simulink library "v2x_modem"  (R2021b)
settings: Solver=VariableStepAuto  StartTime=0.0  StopTime=10.0  RelTol=1e-3
libraries: commsync2 x3, commrfcorlib x2, commfilt2 x2, dspstat3 x1, commrflib2 x1
settings Model: Creator=jacob  LastModifiedBy=jacob

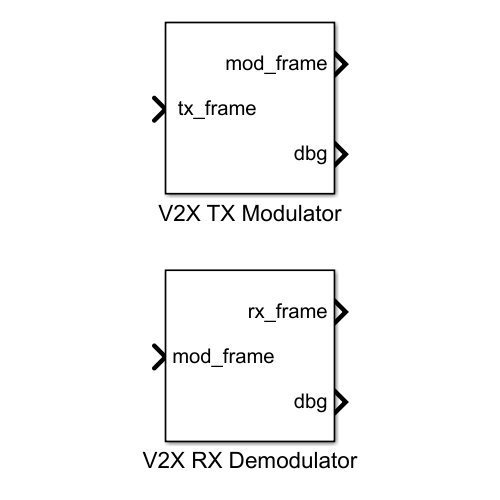
[thumbnail: Simulink's stored preview of the top-level diagram]
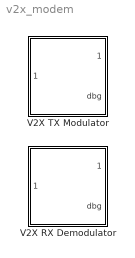
== system v2x_modem ==
  V2X RX Demodulator : Subsystem
      mask init:
      | ini = v2x_modem_init();
  V2X TX Modulator : Subsystem
      mask init:
      | ini = v2x_modem_init();

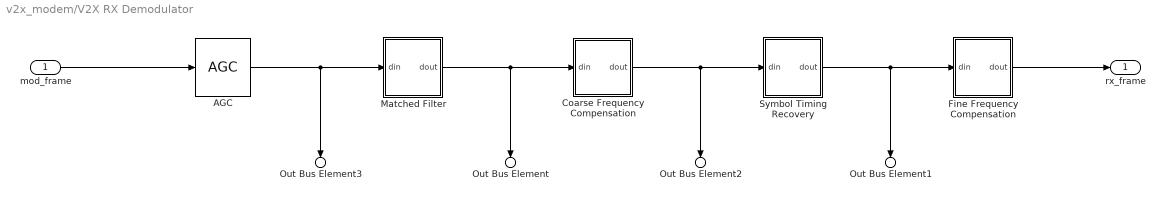
== system v2x_modem/V2X RX Demodulator ==
  mod_frame : Inport
  AGC : commrfcorlib/AGC  LegacyMode=off  DetectorMethod=Rectifier  LoopMethod=Linear  UpdatePeriod=100  StepSize=0.1  AdaptationStepSize=ini.agc_params.step_size  DesiredOutputPower=ini.agc_params.desired_out_pwr  AveragingLength=ini.agc_params.avg_len  MaximumGain=30  MaxPowerGain=ini.agc_params.max_gain_dB  GainOutputPort=off  InputPowerOutputPort=off  SimulateUsing=Interpreted execution
  Coarse Frequency Compensation : Subsystem
  Fine Frequency Compensation : Subsystem
  Matched Filter : Subsystem
  Symbol Timing Recovery : Subsystem
  rx_frame : Outport
  Out Bus Element3 : Outport  Port=2  PortName=dbg  Element=agc_out
  Out Bus Element : Outport  Port=2  PortName=dbg  Element=mf_out
  Out Bus Element2 : Outport  Port=2  PortName=dbg  Element=cfc_out
  Out Bus Element1 : Outport  Port=2  PortName=dbg  Element=str_out
  wires:
  AGC/1 -> Matched Filter/1(din), Out Bus Element3/1
  Coarse Frequency Compensation/1(dout) -> Out Bus Element2/1, Symbol Timing Recovery/1(din)
  Fine Frequency Compensation/1(dout) -> rx_frame/1
  Symbol Timing Recovery/1(dout) -> Out Bus Element1/1, Fine Frequency Compensation/1(din)
  Matched Filter/1(dout) -> Coarse Frequency Compensation/1(din), Out Bus Element/1
  mod_frame/1 -> AGC/1

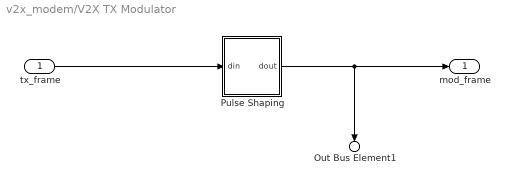
== system v2x_modem/V2X TX Modulator ==
  " tx_frame" : Inport
  Pulse Shaping : Subsystem
  mod_frame : Outport
  Out Bus Element1 : Outport  Port=2  PortName=dbg  Element=ps_out
  wires:
  " tx_frame"/1 -> Pulse Shaping/1(din)
  Pulse Shaping/1(dout) -> Out Bus Element1/1, mod_frame/1

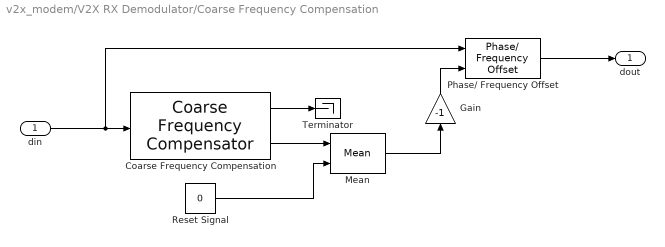
== system v2x_modem/V2X RX Demodulator/Coarse Frequency Compensation ==
  din : Inport
  Coarse Frequency Compensation : commrfcorlib/Coarse Frequency Compensator  Modulation=QPSK  Algorithm=Correlation-based  FrequencyResolution=25  MaximumFrequencyOffset=ini.freq_params.max_fo  SamplesPerSymbol=4  EstimatedFreqOffsetPort=on  SimulateUsing=Code generation
      settings: SourceProductBaseCode=CM
  Gain : Gain  Gain=-1
  Mean : dspstat3/Mean  run=on  InputProcessing=Columns as channels (frame based)  reset_popup=Either edge  directionMode=Each column  dimension=1  roiEnable=off  roiType=Rectangles  roiPortion=Entire ROI  roiOutput=Individual statistics for each ROI  roiFlag=off  roundingMode=Floor  overflowMode=off  outputDataTypeStr=Inherit: Same as accumulator  outputMin=[]  outputMax=[]  outputLastDataTypeStr=Inherit: Same as accumulator
  Phase/ Frequency Offset : commrflib2/Phase// Frequency Offset  phaseOffset=0  freqPort=on  freqOffset=0
  Reset Signal : Constant  Value=0  SampleTime=-1
  Terminator : Terminator
  dout : Outport  VectorParamsAs1DForOutWhenUnconnected=off
  wires:
  Reset Signal/1 -> Mean/2
  Gain/1 -> Phase/ Frequency Offset/2
  Coarse Frequency Compensation/1 -> Terminator/1
  Coarse Frequency Compensation/2 -> Mean/1
  Mean/1 -> Gain/1
  Phase/ Frequency Offset/1 -> dout/1
  din/1 -> Coarse Frequency Compensation/1, Phase/ Frequency Offset/1

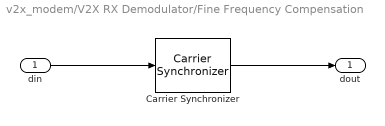
== system v2x_modem/V2X RX Demodulator/Fine Frequency Compensation ==
  din : Inport
  Carrier Synchronizer : commsync2/Carrier Synchronizer  Modulation=QPSK  ModulationPhaseOffset=Auto  CustomPhaseOffset=0  SamplesPerSymbol=ini.srrc_params.sps  DampingFactor=ini.timing_recov_params.damping_fact  NormalizedLoopBandwidth=ini.timing_recov_params.norm_loop_bw  EstimatedPhaseErrorOutputPort=off  SimulateUsing=Code generation
  dout : Outport
  wires:
  Carrier Synchronizer/1 -> dout/1
  din/1 -> Carrier Synchronizer/1

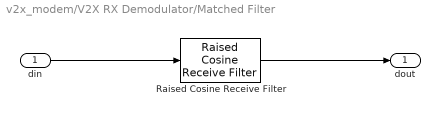
== system v2x_modem/V2X RX Demodulator/Matched Filter ==
  din : Inport
  Raised Cosine Receive Filter : commfilt2/Raised Cosine Receive Filter  filtType=Square root  R=ini.srrc_params.rolloff  filtSpan=ini.srrc_params.filt_span  N=ini.srrc_params.sps  downFactor=ini.srrc_params.decim  downOffset=0  filterGain=ini.srrc_params.lin_amp  InputProcessing=Columns as channels (frame based)  RateOptions=Allow multirate processing  framing=Mute  checkCoeff=off  variableName=rcRxFilt  currentFiltSpan=10  D=5  inputOffset=0  sampMode=Mute  saveAsFlag=0  rateMode=Downsampling  checkGain=Normalized  launchFVT=on  roundingMode=Floor  overflowMode=off  coeffDataTypeStr=Inherit: Same word length as input  coeffMin=[]  coeffMax=[]  coeffLastDataTypeStr=Inherit: Same word length as input  accumDataTypeStr=Inherit: Same as product output  accumLastDataTypeStr=Inherit: Same as product output  outputDataTypeStr=Inherit: Same as accumulator  outputMin=[]  outputMax=[]  outputLastDataTypeStr=Inherit: Same as accumulator
  dout : Outport
  wires:
  Raised Cosine Receive Filter/1 -> dout/1
  din/1 -> Raised Cosine Receive Filter/1

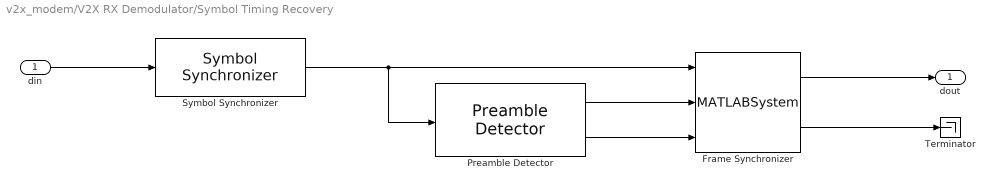
== system v2x_modem/V2X RX Demodulator/Symbol Timing Recovery ==
  din : Inport
  Frame Synchronizer : MATLABSystem  System=FrameSynchronizer  Input=Symbol  OutputFrameLength=ini.bb.intfc_params.tx_frame_len  PreambleLength=ini.bb.preamble_params.len  SimulateUsing=Code generation
      mask Type: FrameSynchronizer
      mask Display:
      | disp(['Frame' char(10) 'Synchronizer']);
      | port_label('input',1,'u');
      | port_label('input',2,'idx');
      | port_label('input',3,'dtMt');
      | port_label('output',1,'Frame');
      | port_label('output',2,'Valid');
  Preamble Detector : commsync2/Preamble Detector  Input=Symbol  Preamble=ini.bb.preamble_params.seq  Threshold=ini.bb.preamble_params.thresh  DetectionMetricOutput=on  Detections=All  SimulateUsing=Interpreted execution
      settings: SourceProductBaseCode=CM
  Symbol Synchronizer : commsync2/Symbol Synchronizer  Modulation=PAM/PSK/QAM  TimingErrorDetector=Early-Late (non-data-aided)  SamplesPerSymbol=ini.srrc_params.sps  DampingFactor=ini.timing_recov_params.damping_fact  NormalizedLoopBandwidth=ini.timing_recov_params.norm_loop_bw  DetectorGain=ini.timing_recov_params.detector_gain  TimingErrorOutputPort=off  SimulateUsing=Code generation
      settings: SourceProductBaseCode=CM
  Terminator : Terminator
  dout : Outport
  wires:
  din/1 -> Symbol Synchronizer/1
  Frame Synchronizer/2 -> Terminator/1
  Frame Synchronizer/1 -> dout/1
  Preamble Detector/2 -> Frame Synchronizer/3
  Preamble Detector/1 -> Frame Synchronizer/2
  Symbol Synchronizer/1 -> Frame Synchronizer/1, Preamble Detector/1

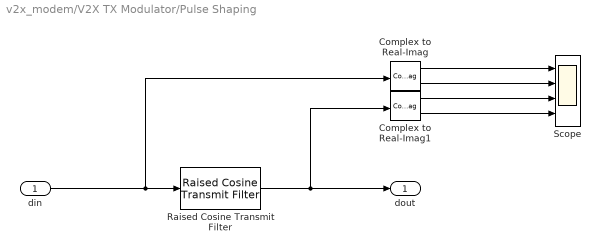
== system v2x_modem/V2X TX Modulator/Pulse Shaping ==
  din : Inport
  Complex to Real-Imag : ComplexToRealImag
  Complex to Real-Imag1 : ComplexToRealImag
  Raised Cosine Transmit Filter : commfilt2/Raised Cosine Transmit Filter  filtType=Square root  R=ini.srrc_params.rolloff  filtSpan=ini.srrc_params.filt_span  N=ini.srrc_params.sps  filterGain=ini.srrc_params.lin_amp  InputProcessing=Columns as channels (frame based)  RateOptions=Enforce single-rate processing  framing=Mute  checkCoeff=off  variableName=rcTxFilt1  checkGain=Normalized  sampMode=Mute  saveAsFlag=0  currentFiltSpan=10  D=(10)/2  launchFVT=on  roundingMode=Floor  overflowMode=off  coeffDataTypeStr=Inherit: Same word length as input  coeffMin=[]  coeffMax=[]  coeffLastDataTypeStr=Inherit: Same word length as input  outputDataTypeStr=Inherit: Same as accumulator  outputMin=[]  outputMax=[]  outputLastDataTypeStr=Inherit: Same as accumulator
  Scope : Scope  NumInputPorts=4
  dout : Outport
  wires:
  din/1 -> Complex to Real-Imag/1, Raised Cosine Transmit Filter/1
  Raised Cosine Transmit Filter/1 -> Complex to Real-Imag1/1, dout/1
  Complex to Real-Imag/1 -> Scope/1
  Complex to Real-Imag/2 -> Scope/2
  Complex to Real-Imag1/1 -> Scope/3
  Complex to Real-Imag1/2 -> Scope/4
